simulink model "sltestProjectorController"  (R2018a)
settings: Solver=FixedStepDiscrete  StartTime=0.0  StopTime=10.0  FixedStep=0.1  RelTol=1e-3  EnableMultiTasking=on
libraries: sltestProjectorCtrlLibrary x1
settings Model: Creator=The MathWorks, Inc.  LastModifiedBy=The MathWorks, Inc.
settings DataIOCC: LimitDataPoints=on  SaveFormat=StructureWithTime  SaveOutput=off  DSMLogging=off  SaveTime=off
settings OptimizationCC: BlockReduction=off  OptimizeBlockIOStorage=off  BufferReuse=off  GlobalBufferReuse=off  ExpressionFolding=off  LocalBlockOutputs=off  LifeSpan=inf
settings DebuggingCC: InheritedTsInSrcMsg=none  AllowSymbolicDim=off  SFUnusedDataAndEventsDiag=none  SFUnexpectedBacktrackingDiag=warning  SFNoUnconditionalDefaultTransitionDiag=none  SFUnreachableExecutionPathDiag=none  SFExecutionAtInitializationDiag=none
settings HardwareCC: ProdBitPerPointer=32  ProdBitPerSizeT=32  ProdBitPerPtrDiffT=32  ProdLargestAtomicFloat=None  ProdWordSize=32  ProdLongLongMode=on  ProdHWDeviceType=Generic->32-bit x86 compatible
settings ModelReferenceCC: PropagateSignalLabelsOutOfModel=off
settings RTWCC: SystemTargetFile=slrt.tlc  TemplateMakefile=slrt_default_tmf  Description=Simulink Real-Time  CodeExecutionProfiling=on  RTWCompilerOptimization=on
settings CodeAppCC: StateflowObjectComments=on
settings ConfigComp: CovMetricSettings=dw  CovHtmlReporting=on  CovSaveCumulativeToWorkspaceVar=on  CovSaveSingleToWorkspaceVar=on  CovExternalEMLEnable=off  DVTestSuiteOptimization=CombinedObjectives (Nonlinear Extended)  DVDetectFloatOverflow=off

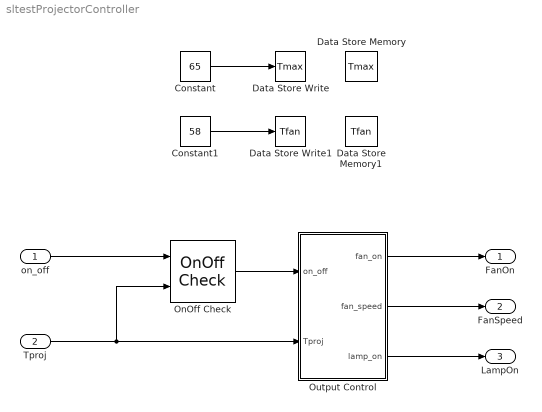
== system sltestProjectorController ==
  on_off : Inport
  Tproj : Inport  Port=2
  Constant : Constant  Value=65  OutDataTypeStr=single
  Constant1 : Constant  Value=58  OutDataTypeStr=single
  Data Store Memory : DataStoreMemory  DataStoreName=Tmax  ReadBeforeWriteMsg=warning  WriteAfterWriteMsg=warning  WriteAfterReadMsg=warning  ShowAdditionalParam=off  OutDataTypeStr=single
  Data Store Memory1 : DataStoreMemory  DataStoreName=Tfan  ReadBeforeWriteMsg=warning  WriteAfterWriteMsg=warning  WriteAfterReadMsg=warning  ShowAdditionalParam=off  OutDataTypeStr=single
  Data Store Write : DataStoreWrite  DataStoreName=Tmax
  Data Store Write1 : DataStoreWrite  DataStoreName=Tfan
  OnOff Check : sltestProjectorCtrlLibrary/OnOff Check
      settings: SourceProductName=Simulink Test  SourceProductBaseCode=SZ
  Output Control : Stateflow chart  RequirementInfo="{}  %GIDa_4f8dcdc0_e872_4bc0_8461_5dd1329f508d"  TreatAsAtomicUnit=on
  FanOn : Outport
  FanSpeed : Outport  Port=2
  LampOn : Outport  Port=3
  wires:
  Constant/1 -> Data Store Write/1
  Constant1/1 -> Data Store Write1/1
  Output Control/1(fan_on) -> FanOn/1
  Output Control/2(fan_speed) -> FanSpeed/1
  Output Control/3(lamp_on) -> LampOn/1
  on_off/1 -> OnOff Check/1
  Tproj/1 -> OnOff Check/2, Output Control/2(Tproj)
  OnOff Check/1 -> Output Control/1(on_off)

== stateflow chart sltestProjectorController/Output Control ==
  state Standby
    entry: fan_on = false;
    lamp_on = false;
    state Switch_off
    state Switch_on
    (default) -> Standby.Switch_off [order 1]
    (default) -> Standby.Switch_on [order 2] : [on_off == 1]
    Standby.Switch_off -> Standby.Switch_on : [on_off == 1]
    Standby.Switch_on -> Standby.Switch_off [order 1] : [on_off == 0]
  state Overheat
    entry: lamp_on = false;
    fan_speed = High
  state Running
    state Projecting_normal
      entry:lamp_on = true;
      state Switch_on
      state Switch_off
      (default) -> Running.Projecting_normal.Switch_on
      Running.Projecting_normal.Switch_on -> Running.Projecting_normal.Switch_off : [on_off == 1]
      Running.Projecting_normal.Switch_off -> Running.Projecting_normal.Switch_on [order 1] : [on_off == 0]
    state Fan_on
      entry: fan_on  = true;
      fan_speed = Low;
    state Projecting_hot
      entry: fan_speed = High;
      state Switch_on1
      state Switch_off
      (default) -> Switch_on1
      Switch_on1 -> Running.Projecting_hot.Switch_off : [on_off == 1]
      Running.Projecting_hot.Switch_off -> Switch_on1 [order 1] : [on_off == 0]
    (default) -> Fan_on
    Fan_on -> (junction 15) : after(2,sec)
    (junction 15) -> Projecting_normal [order 1] : [Tproj < Tfan]
    (junction 15) -> Projecting_hot [order 2]
    Projecting_normal -> Projecting_hot : [Tproj >= Tfan]
    Projecting_hot -> Projecting_normal : after(10,sec)[Tproj < Tfan]
  (default) -> Standby
  Overheat -> Standby : after(15,sec)
  Running.Projecting_hot.Switch_off -> Standby [order 2] : after(2,sec)
  Running.Projecting_normal.Switch_off -> Standby [order 2] : after(2,sec)
  Standby.Switch_on -> Running [order 2] : after(0.5,sec)
  Running -> Overheat : [Tproj >= Tmax]
  data: on_off input boolean size=1; Tproj input single size=1 [0..100]; fan_on output boolean size=1; fan_speed output Enum: FanSpeed size=1; lamp_on output boolean size=1; Tmax data_store_memory; Tfan data_store_memory
